simulink model "PhysicalHyperCook"  (R2026a)
settings: Solver=VariableStepAuto  StopTime=14400
undefined symbols (not defined in the file): Fault_T_Cook1, Fault_T_Cook2, Fault_T_Cook3, Fault_T_Cook4, Fault_T_Pack, Fault_T_Prep1, Fault_T_Prep2, Fault_T_QC, HC_PackRate_bph, HC_PrepRate_bph, HC_QCRate_bph, HC_Resupply_bph, Recipe_Block_s, Recipe_Count, Recipe_Flush_s, Resupply_Cutoff_T, Transport_Latency_s, Transport_Rate_bph
(part 1 of 2)
settings Model: DataDictionary=PhysicalHyperCookData.sldd  Creator=sarah  LastModifiedBy=sdagen

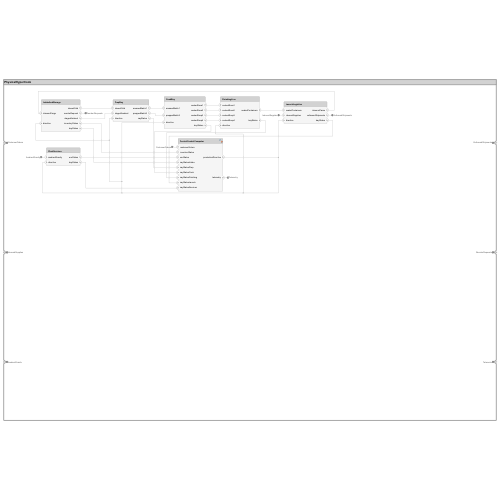
[thumbnail: Simulink's stored preview of the top-level diagram]
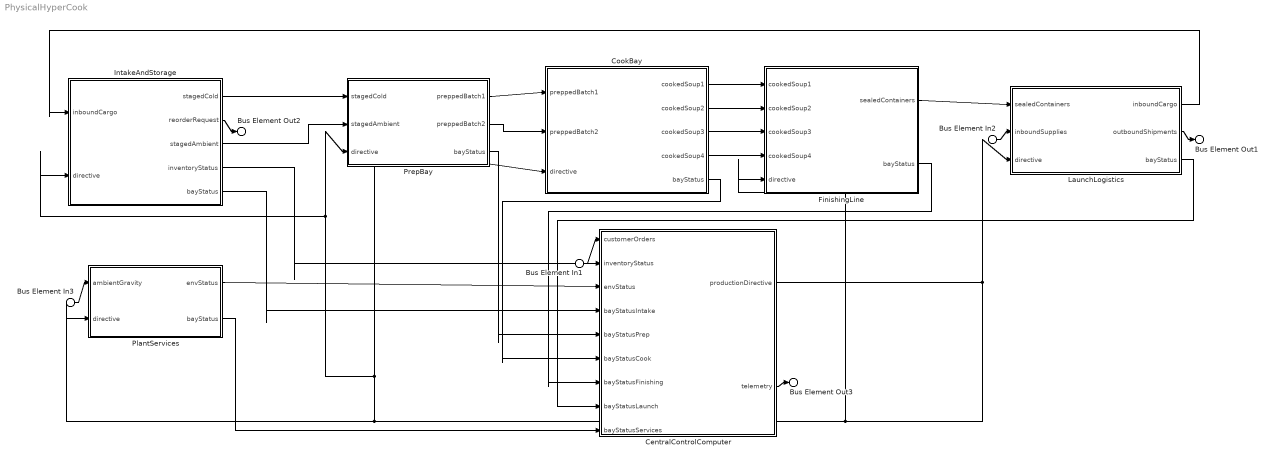
== system PhysicalHyperCook ==
  Bus Element In1 : Inport  PortName=CustomerOrders
  Bus Element In2 : Inport  Port=2  PortName=InboundSupplies
  Bus Element In3 : Inport  Port=3  PortName=AmbientGravity
  CentralControlComputer : Subsystem
      settings: PortSchema="{\"entries\":[{\"content\":{\"headerSize\":26,\"margin\":15,\"minimumSpacing\":25,\"sides\":[{\"content\":{\"connectorIds\":[\"In1\",\"In2\",\"In3\",\"In4\",\"In5\",\"In6\",\"In7\",\"In8\",\"In9\"]},\"type\":\"ConnectorPlacement.EquallySpacedRectSide\",\"uuid\":\"f830f98a-8e8b-4468-adf4-d6eab644987f\"},{\"content\":{\"connectorIds\":[\"Out1\",\"Out2\"],\"side\":\"RIGHT\"},\"type\":\"ConnectorPlacement.EquallySpacedRectSide\",\"uuid\":\"7e0d0116-b3ba-4668-b638-30d0f54ba087\"},{\"content\":{\"side\":\"TOP\"},\"type\":\"ConnectorPlacement.EquallySpacedRectSide\",\"uuid\":\"7b4146d3-46d2-45ca-8c34-b106f0d8cedd\"}]},\"type\":\"ConnectorPlacement.EquallySpacedConnector\",\"uuid\":\"3d911b2d-a78f-42ea-b869-5e09982d9f54\"}],\"packageUris\":[\"http://schema.mathworks.com/mf0/Connector/R2020b\"],\"version\":\"1.0\"}"
  CookBay : Subsystem
      settings: PortSchema="{\"entries\":[{\"content\":{\"headerSize\":26,\"margin\":15,\"minimumSpacing\":25,\"sides\":[{\"content\":{\"connectorIds\":[\"In2\",\"In3\",\"In1\"]},\"type\":\"ConnectorPlacement.EquallySpacedRectSide\",\"uuid\":\"3a94c7fc-0b9e-4df5-a2de-1d2483378dcb\"},{\"content\":{\"connectorIds\":[\"Out1\",\"Out2\",\"Out3\",\"Out4\",\"Out5\"],\"side\":\"RIGHT\"},\"type\":\"ConnectorPlacement.EquallySpacedRectSide\",\"uuid\":\"607e1f04-41cc-4c9a-b401-96cdf33819d0\"},{\"content\":{\"side\":\"TOP\"},\"type\":\"ConnectorPlacement.EquallySpacedRectSide\",\"uuid\":\"2ee07fc7-54c6-4cee-9888-3f37ad01f332\"}]},\"type\":\"ConnectorPlacement.EquallySpacedConnector\",\"uuid\":\"f91f3af9-eaeb-4625-ae6e-5ceb7fb8b64c\"}],\"packageUris\":[\"http://schema.mathworks.com/mf0/Connector/R2020b\"],\"version\":\"1.0\"}"
  FinishingLine : Subsystem
      settings: PortSchema="{\"entries\":[{\"content\":{\"headerSize\":26,\"margin\":15,\"minimumSpacing\":25,\"sides\":[{\"content\":{\"connectorIds\":[\"In2\",\"In3\",\"In4\",\"In5\",\"In1\"]},\"type\":\"ConnectorPlacement.EquallySpacedRectSide\",\"uuid\":\"3a94c7fc-0b9e-4df5-a2de-1d2483378dcb\"},{\"content\":{\"connectorIds\":[\"Out1\",\"Out2\"],\"side\":\"RIGHT\"},\"type\":\"ConnectorPlacement.EquallySpacedRectSide\",\"uuid\":\"607e1f04-41cc-4c9a-b401-96cdf33819d0\"},{\"content\":{\"side\":\"TOP\"},\"type\":\"ConnectorPlacement.EquallySpacedRectSide\",\"uuid\":\"2ee07fc7-54c6-4cee-9888-3f37ad01f332\"}]},\"type\":\"ConnectorPlacement.EquallySpacedConnector\",\"uuid\":\"f91f3af9-eaeb-4625-ae6e-5ceb7fb8b64c\"}],\"packageUris\":[\"http://schema.mathworks.com/mf0/Connector/R2020b\"],\"version\":\"1.0\"}"
  IntakeAndStorage : Subsystem
      settings: PortSchema="{\"entries\":[{\"content\":{\"headerSize\":26,\"margin\":15,\"minimumSpacing\":25,\"sides\":[{\"content\":{\"connectorIds\":[\"In2\",\"In1\"]},\"type\":\"ConnectorPlacement.EquallySpacedRectSide\",\"uuid\":\"3a94c7fc-0b9e-4df5-a2de-1d2483378dcb\"},{\"content\":{\"connectorIds\":[\"Out1\",\"Out2\",\"Out4\",\"Out3\",\"Out5\"],\"side\":\"RIGHT\"},\"type\":\"ConnectorPlacement.EquallySpacedRectSide\",\"uuid\":\"607e1f04-41cc-4c9a-b401-96cdf33819d0\"},{\"content\":{\"side\":\"TOP\"},\"type\":\"ConnectorPlacement.EquallySpacedRectSide\",\"uuid\":\"2ee07fc7-54c6-4cee-9888-3f37ad01f332\"}]},\"type\":\"ConnectorPlacement.EquallySpacedConnector\",\"uuid\":\"f91f3af9-eaeb-4625-ae6e-5ceb7fb8b64c\"}],\"packageUris\":[\"http://schema.mathworks.com/mf0/Connector/R2020b\"],\"version\":\"1.0\"}"
  LaunchLogistics : Subsystem
      settings: PortSchema="{\"entries\":[{\"content\":{\"headerSize\":26,\"margin\":15,\"minimumSpacing\":25,\"sides\":[{\"content\":{\"connectorIds\":[\"In2\",\"In3\",\"In1\"]},\"type\":\"ConnectorPlacement.EquallySpacedRectSide\",\"uuid\":\"3a94c7fc-0b9e-4df5-a2de-1d2483378dcb\"},{\"content\":{\"connectorIds\":[\"Out1\",\"Out2\",\"Out3\"],\"side\":\"RIGHT\"},\"type\":\"ConnectorPlacement.EquallySpacedRectSide\",\"uuid\":\"607e1f04-41cc-4c9a-b401-96cdf33819d0\"},{\"content\":{\"side\":\"TOP\"},\"type\":\"ConnectorPlacement.EquallySpacedRectSide\",\"uuid\":\"2ee07fc7-54c6-4cee-9888-3f37ad01f332\"}]},\"type\":\"ConnectorPlacement.EquallySpacedConnector\",\"uuid\":\"f91f3af9-eaeb-4625-ae6e-5ceb7fb8b64c\"}],\"packageUris\":[\"http://schema.mathworks.com/mf0/Connector/R2020b\"],\"version\":\"1.0\"}"
  PlantServices : Subsystem
      settings: PortSchema="{\"entries\":[{\"content\":{\"headerSize\":26,\"margin\":15,\"minimumSpacing\":25,\"sides\":[{\"content\":{\"connectorIds\":[\"In2\",\"In1\"]},\"type\":\"ConnectorPlacement.EquallySpacedRectSide\",\"uuid\":\"3a94c7fc-0b9e-4df5-a2de-1d2483378dcb\"},{\"content\":{\"connectorIds\":[\"Out1\",\"Out2\"],\"side\":\"RIGHT\"},\"type\":\"ConnectorPlacement.EquallySpacedRectSide\",\"uuid\":\"607e1f04-41cc-4c9a-b401-96cdf33819d0\"},{\"content\":{\"side\":\"TOP\"},\"type\":\"ConnectorPlacement.EquallySpacedRectSide\",\"uuid\":\"2ee07fc7-54c6-4cee-9888-3f37ad01f332\"}]},\"type\":\"ConnectorPlacement.EquallySpacedConnector\",\"uuid\":\"f91f3af9-eaeb-4625-ae6e-5ceb7fb8b64c\"}],\"packageUris\":[\"http://schema.mathworks.com/mf0/Connector/R2020b\"],\"version\":\"1.0\"}"
  PrepBay : Subsystem
      settings: PortSchema="{\"entries\":[{\"content\":{\"headerSize\":26,\"margin\":15,\"minimumSpacing\":25,\"sides\":[{\"content\":{\"connectorIds\":[\"In2\",\"In3\",\"In1\"]},\"type\":\"ConnectorPlacement.EquallySpacedRectSide\",\"uuid\":\"3a94c7fc-0b9e-4df5-a2de-1d2483378dcb\"},{\"content\":{\"connectorIds\":[\"Out1\",\"Out2\",\"Out3\"],\"side\":\"RIGHT\"},\"type\":\"ConnectorPlacement.EquallySpacedRectSide\",\"uuid\":\"607e1f04-41cc-4c9a-b401-96cdf33819d0\"},{\"content\":{\"side\":\"TOP\"},\"type\":\"ConnectorPlacement.EquallySpacedRectSide\",\"uuid\":\"2ee07fc7-54c6-4cee-9888-3f37ad01f332\"}]},\"type\":\"ConnectorPlacement.EquallySpacedConnector\",\"uuid\":\"f91f3af9-eaeb-4625-ae6e-5ceb7fb8b64c\"}],\"packageUris\":[\"http://schema.mathworks.com/mf0/Connector/R2020b\"],\"version\":\"1.0\"}"
  Bus Element Out1 : Outport  PortName=OutboundShipments
  Bus Element Out2 : Outport  Port=2  PortName=ReorderRequests
  Bus Element Out3 : Outport  Port=3  PortName=Telemetry
  wires:
  PrepBay/3(bayStatus) -> CentralControlComputer/5(bayStatusPrep)
  Bus Element In2/1 -> LaunchLogistics/3(inboundSupplies)
  CentralControlComputer/1(productionDirective) -> LaunchLogistics/1(directive), IntakeAndStorage/1(directive), PrepBay/1(directive), CookBay/1(directive), PlantServices/1(directive), FinishingLine/1(directive)
  Bus Element In3/1 -> PlantServices/2(ambientGravity)
  LaunchLogistics/1(inboundCargo) -> IntakeAndStorage/2(inboundCargo)
  LaunchLogistics/2(outboundShipments) -> Bus Element Out1/1
  LaunchLogistics/3(bayStatus) -> CentralControlComputer/8(bayStatusLaunch)
  PrepBay/1(preppedBatch1) -> CookBay/2(preppedBatch1)
  PrepBay/2(preppedBatch2) -> CookBay/3(preppedBatch2)
  FinishingLine/1(sealedContainers) -> LaunchLogistics/2(sealedContainers)
  FinishingLine/2(bayStatus) -> CentralControlComputer/7(bayStatusFinishing)
  IntakeAndStorage/1(stagedCold) -> PrepBay/2(stagedCold)
  IntakeAndStorage/2(reorderRequest) -> Bus Element Out2/1
  IntakeAndStorage/3(inventoryStatus) -> CentralControlComputer/2(inventoryStatus)
  IntakeAndStorage/4(stagedAmbient) -> PrepBay/3(stagedAmbient)
  IntakeAndStorage/5(bayStatus) -> CentralControlComputer/4(bayStatusIntake)
  Bus Element In1/1 -> CentralControlComputer/1(customerOrders)
  CookBay/1(cookedSoup1) -> FinishingLine/2(cookedSoup1)
  CookBay/2(cookedSoup2) -> FinishingLine/3(cookedSoup2)
  CookBay/3(cookedSoup3) -> FinishingLine/4(cookedSoup3)
  CookBay/4(cookedSoup4) -> FinishingLine/5(cookedSoup4)
  CookBay/5(bayStatus) -> CentralControlComputer/6(bayStatusCook)
  PlantServices/2(bayStatus) -> CentralControlComputer/9(bayStatusServices)
  PlantServices/1(envStatus) -> CentralControlComputer/3(envStatus)
  CentralControlComputer/2(telemetry) -> Bus Element Out3/1

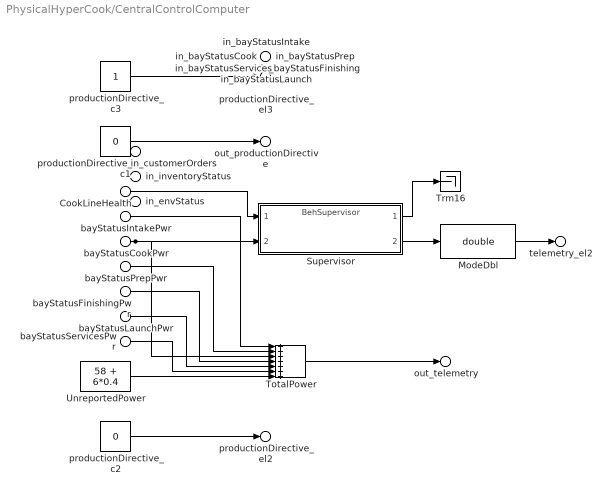
== system PhysicalHyperCook/CentralControlComputer ==
  in_customerOrders : Inport  PortName=customerOrders
  in_inventoryStatus : Inport  Port=2  PortName=inventoryStatus
  in_envStatus : Inport  Port=3  PortName=envStatus
  in_bayStatusIntake : Inport  Port=4  PortName=bayStatusIntake
  bayStatusIntakePwr : Inport  Port=4  PortName=bayStatusIntake  Element=power_kW
  in_bayStatusPrep : Inport  Port=5  PortName=bayStatusPrep
  bayStatusPrepPwr : Inport  Port=5  PortName=bayStatusPrep  Element=power_kW
  in_bayStatusCook : Inport  Port=6  PortName=bayStatusCook  Element=power_kW
  bayStatusCookPwr : Inport  Port=6  PortName=bayStatusCook  Element=power_kW
  CookLineHealth : Inport  Port=6  PortName=bayStatusCook  Element=lineHealth
  in_bayStatusFinishing : Inport  Port=7  PortName=bayStatusFinishing
  bayStatusFinishingPwr : Inport  Port=7  PortName=bayStatusFinishing  Element=power_kW
  in_bayStatusLaunch : Inport  Port=8  PortName=bayStatusLaunch
  bayStatusLaunchPwr : Inport  Port=8  PortName=bayStatusLaunch  Element=power_kW
  in_bayStatusServices : Inport  Port=9  PortName=bayStatusServices
  bayStatusServicesPwr : Inport  Port=9  PortName=bayStatusServices  Element=power_kW
  ModeDbl : DataTypeConversion  OutDataTypeStr=double  SaturateOnIntegerOverflow=off  RndMeth=Floor
  Supervisor : ModelReference  ModelNameDialog=BehSupervisor  ParameterArgumentNames=NumLines  ParameterArgumentValues=HC_NumLines  UsingDefaultArgumentValue=0  SimulationMode=Normal  ModelReferenceVersion=1.8
  TotalPower : Sum  Inputs=+++++++
  Trm16 : Terminator
  UnreportedPower : Constant  Value=58 + 6*0.4
  productionDirective_c1 : Constant  Value=0
  productionDirective_c2 : Constant  Value=0
  productionDirective_c3 : Constant
  out_productionDirective : Outport  PortName=productionDirective  Element=cmdType
  productionDirective_el2 : Outport  PortName=productionDirective  Element=targetId
  productionDirective_el3 : Outport  PortName=productionDirective  Element=setpoint
  out_telemetry : Outport  Port=2  PortName=telemetry  Element=totalPower_kW
  telemetry_el2 : Outport  Port=2  PortName=telemetry  Element=plantMode
  wires:
  productionDirective_c3/1 -> productionDirective_el3/1
  bayStatusPrepPwr/1 -> TotalPower/2
  CookLineHealth/1 -> Supervisor/1
  productionDirective_c1/1 -> out_productionDirective/1
  bayStatusIntakePwr/1 -> TotalPower/1
  bayStatusLaunchPwr/1 -> TotalPower/5
  bayStatusCookPwr/1 -> Supervisor/2, TotalPower/3
  bayStatusFinishingPwr/1 -> TotalPower/4
  Supervisor/2 -> ModeDbl/1
  bayStatusServicesPwr/1 -> TotalPower/6
  UnreportedPower/1 -> TotalPower/7
  productionDirective_c2/1 -> productionDirective_el2/1
  Supervisor/1 -> Trm16/1
  TotalPower/1 -> out_telemetry/1
  ModeDbl/1 -> telemetry_el2/1

== system PhysicalHyperCook/CookBay ==
  Bus Element In1 : Inport  PortName=directive
  Bus Element In3 : Inport  Port=2  PortName=preppedBatch1
  Bus Element In4 : Inport  Port=3  PortName=preppedBatch2
  ContinuousCookLine1 : Subsystem
      settings: PortSchema="{\"entries\":[{\"content\":{\"headerSize\":26,\"margin\":15,\"minimumSpacing\":25,\"sides\":[{\"content\":{\"connectorIds\":[\"In1\",\"In2\"]},\"type\":\"ConnectorPlacement.EquallySpacedRectSide\",\"uuid\":\"f830f98a-8e8b-4468-adf4-d6eab644987f\"},{\"content\":{\"connectorIds\":[\"Out1\",\"Out2\"],\"side\":\"RIGHT\"},\"type\":\"ConnectorPlacement.EquallySpacedRectSide\",\"uuid\":\"7e0d0116-b3ba-4668-b638-30d0f54ba087\"},{\"content\":{\"side\":\"TOP\"},\"type\":\"ConnectorPlacement.EquallySpacedRectSide\",\"uuid\":\"7b4146d3-46d2-45ca-8c34-b106f0d8cedd\"}]},\"type\":\"ConnectorPlacement.EquallySpacedConnector\",\"uuid\":\"3d911b2d-a78f-42ea-b869-5e09982d9f54\"}],\"packageUris\":[\"http://schema.mathworks.com/mf0/Connector/R2020b\"],\"version\":\"1.0\"}"
  ContinuousCookLine2 : Subsystem
      settings: PortSchema="{\"entries\":[{\"content\":{\"headerSize\":26,\"margin\":15,\"minimumSpacing\":25,\"sides\":[{\"content\":{\"connectorIds\":[\"In1\",\"In2\"]},\"type\":\"ConnectorPlacement.EquallySpacedRectSide\",\"uuid\":\"f830f98a-8e8b-4468-adf4-d6eab644987f\"},{\"content\":{\"connectorIds\":[\"Out1\",\"Out2\"],\"side\":\"RIGHT\"},\"type\":\"ConnectorPlacement.EquallySpacedRectSide\",\"uuid\":\"7e0d0116-b3ba-4668-b638-30d0f54ba087\"},{\"content\":{\"side\":\"TOP\"},\"type\":\"ConnectorPlacement.EquallySpacedRectSide\",\"uuid\":\"7b4146d3-46d2-45ca-8c34-b106f0d8cedd\"}]},\"type\":\"ConnectorPlacement.EquallySpacedConnector\",\"uuid\":\"3d911b2d-a78f-42ea-b869-5e09982d9f54\"}],\"packageUris\":[\"http://schema.mathworks.com/mf0/Connector/R2020b\"],\"version\":\"1.0\"}"
  ContinuousCookLine3 : Subsystem
      settings: PortSchema="{\"entries\":[{\"content\":{\"headerSize\":26,\"margin\":15,\"minimumSpacing\":25,\"sides\":[{\"content\":{\"connectorIds\":[\"In1\",\"In2\"]},\"type\":\"ConnectorPlacement.EquallySpacedRectSide\",\"uuid\":\"f830f98a-8e8b-4468-adf4-d6eab644987f\"},{\"content\":{\"connectorIds\":[\"Out1\",\"Out2\"],\"side\":\"RIGHT\"},\"type\":\"ConnectorPlacement.EquallySpacedRectSide\",\"uuid\":\"7e0d0116-b3ba-4668-b638-30d0f54ba087\"},{\"content\":{\"side\":\"TOP\"},\"type\":\"ConnectorPlacement.EquallySpacedRectSide\",\"uuid\":\"7b4146d3-46d2-45ca-8c34-b106f0d8cedd\"}]},\"type\":\"ConnectorPlacement.EquallySpacedConnector\",\"uuid\":\"3d911b2d-a78f-42ea-b869-5e09982d9f54\"}],\"packageUris\":[\"http://schema.mathworks.com/mf0/Connector/R2020b\"],\"version\":\"1.0\"}"
  ContinuousCookLine4 : Subsystem
      settings: PortSchema="{\"entries\":[{\"content\":{\"headerSize\":26,\"margin\":15,\"minimumSpacing\":25,\"sides\":[{\"content\":{\"connectorIds\":[\"In1\",\"In2\"]},\"type\":\"ConnectorPlacement.EquallySpacedRectSide\",\"uuid\":\"f830f98a-8e8b-4468-adf4-d6eab644987f\"},{\"content\":{\"connectorIds\":[\"Out1\",\"Out2\"],\"side\":\"RIGHT\"},\"type\":\"ConnectorPlacement.EquallySpacedRectSide\",\"uuid\":\"7e0d0116-b3ba-4668-b638-30d0f54ba087\"},{\"content\":{\"side\":\"TOP\"},\"type\":\"ConnectorPlacement.EquallySpacedRectSide\",\"uuid\":\"7b4146d3-46d2-45ca-8c34-b106f0d8cedd\"}]},\"type\":\"ConnectorPlacement.EquallySpacedConnector\",\"uuid\":\"3d911b2d-a78f-42ea-b869-5e09982d9f54\"}],\"packageUris\":[\"http://schema.mathworks.com/mf0/Connector/R2020b\"],\"version\":\"1.0\"}"
  CookController : Subsystem
      settings: PortSchema="{\"entries\":[{\"content\":{\"headerSize\":26,\"margin\":15,\"minimumSpacing\":25,\"sides\":[{\"content\":{\"connectorIds\":[\"In1\",\"In2\",\"In3\",\"In4\",\"In5\"]},\"type\":\"ConnectorPlacement.EquallySpacedRectSide\",\"uuid\":\"0731d988-4a26-4db6-8347-b78d2aa6954f\"},{\"content\":{\"connectorIds\":[\"Out1\",\"Out2\"],\"side\":\"RIGHT\"},\"type\":\"ConnectorPlacement.EquallySpacedRectSide\",\"uuid\":\"6e8ac7ed-a816-4c7e-8f31-c61224c9ac03\"},{\"content\":{\"side\":\"TOP\"},\"type\":\"ConnectorPlacement.EquallySpacedRectSide\",\"uuid\":\"7c48a918-2743-4697-bc21-ce4fb8bbcea2\"}]},\"type\":\"ConnectorPlacement.EquallySpacedConnector\",\"uuid\":\"5e30be34-c1af-4919-9af8-d4df8145ecd1\"}],\"packageUris\":[\"http://schema.mathworks.com/mf0/Connector/R2020b\"],\"version\":\"1.0\"}"
  Bus Element Out5 : Outport  PortName=cookedSoup1
  Bus Element Out6 : Outport  Port=2  PortName=cookedSoup2
  Bus Element Out7 : Outport  Port=3  PortName=cookedSoup3
  Bus Element Out8 : Outport  Port=4  PortName=cookedSoup4
  Bus Element Out9 : Outport  Port=5  PortName=bayStatus
  wires:
  Bus Element In1/1 -> CookController/1(directive)
  CookController/2(bayStatus) -> Bus Element Out9/1
  ContinuousCookLine4/2(statusCook4) -> CookController/5(statusCook4)
  Bus Element In3/1 -> ContinuousCookLine1/1(preppedBatch1), ContinuousCookLine2/1(preppedBatch1)
  CookController/1(bayDirective) -> ContinuousCookLine1/2(directive), ContinuousCookLine3/2(directive), ContinuousCookLine2/2(directive), ContinuousCookLine4/2(directive)
  Bus Element In4/1 -> ContinuousCookLine4/1(preppedBatch2), ContinuousCookLine3/1(preppedBatch2)
  ContinuousCookLine4/1(cookedSoup4) -> Bus Element Out8/1
  ContinuousCookLine2/1(cookedSoup2) -> Bus Element Out6/1
  ContinuousCookLine2/2(statusCook2) -> CookController/3(statusCook2)
  ContinuousCookLine1/1(cookedSoup1) -> Bus Element Out5/1
  ContinuousCookLine1/2(statusCook1) -> CookController/2(statusCook1)
  ContinuousCookLine3/1(cookedSoup3) -> Bus Element Out7/1
  ContinuousCookLine3/2(statusCook3) -> CookController/4(statusCook3)

== system PhysicalHyperCook/FinishingLine ==
  Bus Element In1 : Inport  PortName=directive
  Bus Element In3 : Inport  Port=2  PortName=cookedSoup1
  Bus Element In4 : Inport  Port=3  PortName=cookedSoup2
  Bus Element In5 : Inport  Port=4  PortName=cookedSoup3
  Bus Element In6 : Inport  Port=5  PortName=cookedSoup4
  FinishingController : Subsystem
      settings: PortSchema="{\"entries\":[{\"content\":{\"headerSize\":26,\"margin\":15,\"minimumSpacing\":25,\"sides\":[{\"content\":{\"connectorIds\":[\"In1\",\"In2\",\"In3\"]},\"type\":\"ConnectorPlacement.EquallySpacedRectSide\",\"uuid\":\"0731d988-4a26-4db6-8347-b78d2aa6954f\"},{\"content\":{\"connectorIds\":[\"Out1\",\"Out2\"],\"side\":\"RIGHT\"},\"type\":\"ConnectorPlacement.EquallySpacedRectSide\",\"uuid\":\"6e8ac7ed-a816-4c7e-8f31-c61224c9ac03\"},{\"content\":{\"side\":\"TOP\"},\"type\":\"ConnectorPlacement.EquallySpacedRectSide\",\"uuid\":\"7c48a918-2743-4697-bc21-ce4fb8bbcea2\"}]},\"type\":\"ConnectorPlacement.EquallySpacedConnector\",\"uuid\":\"5e30be34-c1af-4919-9af8-d4df8145ecd1\"}],\"packageUris\":[\"http://schema.mathworks.com/mf0/Connector/R2020b\"],\"version\":\"1.0\"}"
  HighSpeedPackagingLine : Subsystem
      settings: PortSchema="{\"entries\":[{\"content\":{\"headerSize\":26,\"margin\":15,\"minimumSpacing\":25,\"sides\":[{\"content\":{\"connectorIds\":[\"In1\",\"In2\"]},\"type\":\"ConnectorPlacement.EquallySpacedRectSide\",\"uuid\":\"f830f98a-8e8b-4468-adf4-d6eab644987f\"},{\"content\":{\"connectorIds\":[\"Out1\",\"Out2\"],\"side\":\"RIGHT\"},\"type\":\"ConnectorPlacement.EquallySpacedRectSide\",\"uuid\":\"7e0d0116-b3ba-4668-b638-30d0f54ba087\"},{\"content\":{\"side\":\"TOP\"},\"type\":\"ConnectorPlacement.EquallySpacedRectSide\",\"uuid\":\"7b4146d3-46d2-45ca-8c34-b106f0d8cedd\"}]},\"type\":\"ConnectorPlacement.EquallySpacedConnector\",\"uuid\":\"3d911b2d-a78f-42ea-b869-5e09982d9f54\"}],\"packageUris\":[\"http://schema.mathworks.com/mf0/Connector/R2020b\"],\"version\":\"1.0\"}"
  InlineQCScanner : Subsystem
      settings: PortSchema="{\"entries\":[{\"content\":{\"headerSize\":26,\"margin\":15,\"minimumSpacing\":25,\"sides\":[{\"content\":{\"connectorIds\":[\"In1\",\"In2\",\"In3\",\"In4\",\"In5\"]},\"type\":\"ConnectorPlacement.EquallySpacedRectSide\",\"uuid\":\"f830f98a-8e8b-4468-adf4-d6eab644987f\"},{\"content\":{\"connectorIds\":[\"Out1\",\"Out2\"],\"side\":\"RIGHT\"},\"type\":\"ConnectorPlacement.EquallySpacedRectSide\",\"uuid\":\"7e0d0116-b3ba-4668-b638-30d0f54ba087\"},{\"content\":{\"side\":\"TOP\"},\"type\":\"ConnectorPlacement.EquallySpacedRectSide\",\"uuid\":\"7b4146d3-46d2-45ca-8c34-b106f0d8cedd\"}]},\"type\":\"ConnectorPlacement.EquallySpacedConnector\",\"uuid\":\"3d911b2d-a78f-42ea-b869-5e09982d9f54\"}],\"packageUris\":[\"http://schema.mathworks.com/mf0/Connector/R2020b\"],\"version\":\"1.0\"}"
  Bus Element Out1 : Outport  PortName=sealedContainers
  Bus Element Out4 : Outport  Port=2  PortName=bayStatus
  wires:
  Bus Element In3/1 -> InlineQCScanner/1(cookedSoup1)
  Bus Element In4/1 -> InlineQCScanner/2(cookedSoup2)
  Bus Element In5/1 -> InlineQCScanner/3(cookedSoup3)
  Bus Element In6/1 -> InlineQCScanner/4(cookedSoup4)
  HighSpeedPackagingLine/2(statusPack) -> FinishingController/2(statusPack)
  InlineQCScanner/1(approvedSoup) -> HighSpeedPackagingLine/1(approvedSoup)
  HighSpeedPackagingLine/1(sealedContainers) -> Bus Element Out1/1
  InlineQCScanner/2(statusQA) -> FinishingController/3(statusQA)
  Bus Element In1/1 -> FinishingController/1(directive)
  FinishingController/1(bayDirective) -> InlineQCScanner/5(directive), HighSpeedPackagingLine/2(directive)
  FinishingController/2(bayStatus) -> Bus Element Out4/1

== system PhysicalHyperCook/IntakeAndStorage ==
  Bus Element In1 : Inport  PortName=directive
  Bus Element In2 : Inport  Port=2  PortName=inboundCargo
  AmbientStorageSilo : Subsystem
      settings: PortSchema="{\"entries\":[{\"content\":{\"headerSize\":26,\"margin\":15,\"minimumSpacing\":25,\"sides\":[{\"content\":{\"connectorIds\":[\"In1\",\"In2\"]},\"type\":\"ConnectorPlacement.EquallySpacedRectSide\",\"uuid\":\"f830f98a-8e8b-4468-adf4-d6eab644987f\"},{\"content\":{\"connectorIds\":[\"Out1\",\"Out2\",\"Out3\"],\"side\":\"RIGHT\"},\"type\":\"ConnectorPlacement.EquallySpacedRectSide\",\"uuid\":\"7e0d0116-b3ba-4668-b638-30d0f54ba087\"},{\"content\":{\"side\":\"TOP\"},\"type\":\"ConnectorPlacement.EquallySpacedRectSide\",\"uuid\":\"7b4146d3-46d2-45ca-8c34-b106f0d8cedd\"}]},\"type\":\"ConnectorPlacement.EquallySpacedConnector\",\"uuid\":\"3d911b2d-a78f-42ea-b869-5e09982d9f54\"}],\"packageUris\":[\"http://schema.mathworks.com/mf0/Connector/R2020b\"],\"version\":\"1.0\"}"
  CargoGantryDock : Subsystem
      settings: PortSchema="{\"entries\":[{\"content\":{\"headerSize\":26,\"margin\":15,\"minimumSpacing\":25,\"sides\":[{\"content\":{\"connectorIds\":[\"In1\",\"In2\"]},\"type\":\"ConnectorPlacement.EquallySpacedRectSide\",\"uuid\":\"f830f98a-8e8b-4468-adf4-d6eab644987f\"},{\"content\":{\"connectorIds\":[\"Out1\",\"Out2\"],\"side\":\"RIGHT\"},\"type\":\"ConnectorPlacement.EquallySpacedRectSide\",\"uuid\":\"7e0d0116-b3ba-4668-b638-30d0f54ba087\"},{\"content\":{\"side\":\"TOP\"},\"type\":\"ConnectorPlacement.EquallySpacedRectSide\",\"uuid\":\"7b4146d3-46d2-45ca-8c34-b106f0d8cedd\"}]},\"type\":\"ConnectorPlacement.EquallySpacedConnector\",\"uuid\":\"3d911b2d-a78f-42ea-b869-5e09982d9f54\"}],\"packageUris\":[\"http://schema.mathworks.com/mf0/Connector/R2020b\"],\"version\":\"1.0\"}"
  ColdStorageVault : Subsystem
      settings: PortSchema="{\"entries\":[{\"content\":{\"headerSize\":26,\"margin\":15,\"minimumSpacing\":25,\"sides\":[{\"content\":{\"connectorIds\":[\"In1\",\"In2\"]},\"type\":\"ConnectorPlacement.EquallySpacedRectSide\",\"uuid\":\"f830f98a-8e8b-4468-adf4-d6eab644987f\"},{\"content\":{\"connectorIds\":[\"Out1\",\"Out2\",\"Out3\"],\"side\":\"RIGHT\"},\"type\":\"ConnectorPlacement.EquallySpacedRectSide\",\"uuid\":\"7e0d0116-b3ba-4668-b638-30d0f54ba087\"},{\"content\":{\"side\":\"TOP\"},\"type\":\"ConnectorPlacement.EquallySpacedRectSide\",\"uuid\":\"7b4146d3-46d2-45ca-8c34-b106f0d8cedd\"}]},\"type\":\"ConnectorPlacement.EquallySpacedConnector\",\"uuid\":\"3d911b2d-a78f-42ea-b869-5e09982d9f54\"}],\"packageUris\":[\"http://schema.mathworks.com/mf0/Connector/R2020b\"],\"version\":\"1.0\"}"
  IntakeController : Subsystem
      settings: PortSchema="{\"entries\":[{\"content\":{\"headerSize\":26,\"margin\":15,\"minimumSpacing\":25,\"sides\":[{\"content\":{\"connectorIds\":[\"In1\",\"In2\",\"In3\",\"In4\"]},\"type\":\"ConnectorPlacement.EquallySpacedRectSide\",\"uuid\":\"0731d988-4a26-4db6-8347-b78d2aa6954f\"},{\"content\":{\"connectorIds\":[\"Out1\",\"Out2\"],\"side\":\"RIGHT\"},\"type\":\"ConnectorPlacement.EquallySpacedRectSide\",\"uuid\":\"6e8ac7ed-a816-4c7e-8f31-c61224c9ac03\"},{\"content\":{\"side\":\"TOP\"},\"type\":\"ConnectorPlacement.EquallySpacedRectSide\",\"uuid\":\"7c48a918-2743-4697-bc21-ce4fb8bbcea2\"}]},\"type\":\"ConnectorPlacement.EquallySpacedConnector\",\"uuid\":\"5e30be34-c1af-4919-9af8-d4df8145ecd1\"}],\"packageUris\":[\"http://schema.mathworks.com/mf0/Connector/R2020b\"],\"version\":\"1.0\"}"
  InventorySensorGrid : Subsystem
      settings: PortSchema="{\"entries\":[{\"content\":{\"headerSize\":26,\"margin\":15,\"minimumSpacing\":25,\"sides\":[{\"content\":{\"connectorIds\":[\"In1\",\"In2\"]},\"type\":\"ConnectorPlacement.EquallySpacedRectSide\",\"uuid\":\"f830f98a-8e8b-4468-adf4-d6eab644987f\"},{\"content\":{\"connectorIds\":[\"Out1\",\"Out2\"],\"side\":\"RIGHT\"},\"type\":\"ConnectorPlacement.EquallySpacedRectSide\",\"uuid\":\"7e0d0116-b3ba-4668-b638-30d0f54ba087\"},{\"content\":{\"side\":\"TOP\"},\"type\":\"ConnectorPlacement.EquallySpacedRectSide\",\"uuid\":\"7b4146d3-46d2-45ca-8c34-b106f0d8cedd\"}]},\"type\":\"ConnectorPlacement.EquallySpacedConnector\",\"uuid\":\"3d911b2d-a78f-42ea-b869-5e09982d9f54\"}],\"packageUris\":[\"http://schema.mathworks.com/mf0/Connector/R2020b\"],\"version\":\"1.0\"}"
  Bus Element Out1 : Outport  PortName=stagedCold
  Bus Element Out2 : Outport  Port=2  PortName=reorderRequest
  Bus Element Out3 : Outport  Port=3  PortName=inventoryStatus
  Bus Element Out7 : Outport  Port=4  PortName=stagedAmbient
  Bus Element Out8 : Outport  Port=5  PortName=bayStatus
  wires:
  ColdStorageVault/1(stagedCold) -> Bus Element Out1/1
  IntakeController/1(bayDirective) -> AmbientStorageSilo/2(directive), ColdStorageVault/2(directive), CargoGantryDock/2(directive)
  Bus Element In1/1 -> IntakeController/1(directive)
  AmbientStorageSilo/2(stockAmbient) -> InventorySensorGrid/2(stockAmbient)
  Bus Element In2/1 -> CargoGantryDock/1(inboundCargo)
  CargoGantryDock/2(statusReceive) -> IntakeController/3(statusReceive)
  IntakeController/2(bayStatus) -> Bus Element Out8/1
  CargoGantryDock/1(receivedIngredients) -> ColdStorageVault/1(receivedIngredients), AmbientStorageSilo/1(receivedIngredients)
  AmbientStorageSilo/1(stagedAmbient) -> Bus Element Out7/1
  AmbientStorageSilo/3(statusAmbStore) -> IntakeController/2(statusAmbStore)
  ColdStorageVault/3(statusColdStore) -> IntakeController/4(statusColdStore)
  ColdStorageVault/2(stockCold) -> InventorySensorGrid/1(stockCold)
  InventorySensorGrid/1(inventoryStatus) -> Bus Element Out3/1
  InventorySensorGrid/2(reorderRequest) -> Bus Element Out2/1

== system PhysicalHyperCook/LaunchLogistics ==
  Bus Element In1 : Inport  PortName=directive
  Bus Element In2 : Inport  Port=2  PortName=sealedContainers
  Bus Element In4 : Inport  Port=3  PortName=inboundSupplies
  CargoLoaderGantry : Subsystem
      settings: PortSchema="{\"entries\":[{\"content\":{\"headerSize\":26,\"margin\":15,\"minimumSpacing\":25,\"sides\":[{\"content\":{\"connectorIds\":[\"In1\",\"In2\"]},\"type\":\"ConnectorPlacement.EquallySpacedRectSide\",\"uuid\":\"f830f98a-8e8b-4468-adf4-d6eab644987f\"},{\"content\":{\"connectorIds\":[\"Out1\",\"Out2\",\"Out3\"],\"side\":\"RIGHT\"},\"type\":\"ConnectorPlacement.EquallySpacedRectSide\",\"uuid\":\"7e0d0116-b3ba-4668-b638-30d0f54ba087\"},{\"content\":{\"side\":\"TOP\"},\"type\":\"ConnectorPlacement.EquallySpacedRectSide\",\"uuid\":\"7b4146d3-46d2-45ca-8c34-b106f0d8cedd\"}]},\"type\":\"ConnectorPlacement.EquallySpacedConnector\",\"uuid\":\"3d911b2d-a78f-42ea-b869-5e09982d9f54\"}],\"packageUris\":[\"http://schema.mathworks.com/mf0/Connector/R2020b\"],\"version\":\"1.0\"}"
  LaunchController : Subsystem
      settings: PortSchema="{\"entries\":[{\"content\":{\"headerSize\":26,\"margin\":15,\"minimumSpacing\":25,\"sides\":[{\"content\":{\"connectorIds\":[\"In1\",\"In2\",\"In3\",\"In4\"]},\"type\":\"ConnectorPlacement.EquallySpacedRectSide\",\"uuid\":\"0731d988-4a26-4db6-8347-b78d2aa6954f\"},{\"content\":{\"connectorIds\":[\"Out1\",\"Out2\"],\"side\":\"RIGHT\"},\"type\":\"ConnectorPlacement.EquallySpacedRectSide\",\"uuid\":\"6e8ac7ed-a816-4c7e-8f31-c61224c9ac03\"},{\"content\":{\"side\":\"TOP\"},\"type\":\"ConnectorPlacement.EquallySpacedRectSide\",\"uuid\":\"7c48a918-2743-4697-bc21-ce4fb8bbcea2\"}]},\"type\":\"ConnectorPlacement.EquallySpacedConnector\",\"uuid\":\"5e30be34-c1af-4919-9af8-d4df8145ecd1\"}],\"packageUris\":[\"http://schema.mathworks.com/mf0/Connector/R2020b\"],\"version\":\"1.0\"}"
  LaunchPadComplex : Subsystem
      settings: PortSchema="{\"entries\":[{\"content\":{\"headerSize\":26,\"margin\":15,\"minimumSpacing\":25,\"sides\":[{\"content\":{\"connectorIds\":[\"In1\",\"In2\",\"In3\",\"In4\"]},\"type\":\"ConnectorPlacement.EquallySpacedRectSide\",\"uuid\":\"f830f98a-8e8b-4468-adf4-d6eab644987f\"},{\"content\":{\"connectorIds\":[\"Out1\",\"Out2\",\"Out3\"],\"side\":\"RIGHT\"},\"type\":\"ConnectorPlacement.EquallySpacedRectSide\",\"uuid\":\"7e0d0116-b3ba-4668-b638-30d0f54ba087\"},{\"content\":{\"side\":\"TOP\"},\"type\":\"ConnectorPlacement.EquallySpacedRectSide\",\"uuid\":\"7b4146d3-46d2-45ca-8c34-b106f0d8cedd\"}]},\"type\":\"ConnectorPlacement.EquallySpacedConnector\",\"uuid\":\"3d911b2d-a78f-42ea-b869-5e09982d9f54\"}],\"packageUris\":[\"http://schema.mathworks.com/mf0/Connector/R2020b\"],\"version\":\"1.0\"}"
  RefuelingStation : Subsystem
      settings: PortSchema="{\"entries\":[{\"content\":{\"headerSize\":26,\"margin\":15,\"minimumSpacing\":25,\"sides\":[{\"content\":{\"connectorIds\":[\"In1\"]},\"type\":\"ConnectorPlacement.EquallySpacedRectSide\",\"uuid\":\"f830f98a-8e8b-4468-adf4-d6eab644987f\"},{\"content\":{\"connectorIds\":[\"Out1\"],\"side\":\"RIGHT\"},\"type\":\"ConnectorPlacement.EquallySpacedRectSide\",\"uuid\":\"7e0d0116-b3ba-4668-b638-30d0f54ba087\"},{\"content\":{\"side\":\"TOP\"},\"type\":\"ConnectorPlacement.EquallySpacedRectSide\",\"uuid\":\"7b4146d3-46d2-45ca-8c34-b106f0d8cedd\"}]},\"type\":\"ConnectorPlacement.EquallySpacedConnector\",\"uuid\":\"3d911b2d-a78f-42ea-b869-5e09982d9f54\"}],\"packageUris\":[\"http://schema.mathworks.com/mf0/Connector/R2020b\"],\"version\":\"1.0\"}"
  Bus Element Out1 : Outport  PortName=inboundCargo
  Bus Element Out5 : Outport  Port=2  PortName=outboundShipments
  Bus Element Out6 : Outport  Port=3  PortName=bayStatus
  wires:
  LaunchPadComplex/2(outboundShipments) -> Bus Element Out5/1
  LaunchController/1(bayDirective) -> RefuelingStation/1(directive), CargoLoaderGantry/2(directive), LaunchPadComplex/3(directive)
  Bus Element In4/1 -> LaunchPadComplex/4(inboundSupplies)
  Bus Element In2/1 -> CargoLoaderGantry/1(sealedContainers)
  RefuelingStation/1(statusRefuel) -> LaunchController/4(statusRefuel)
  LaunchPadComplex/1(inboundCargo) -> Bus Element Out1/1
  LaunchPadComplex/3(statusFleet) -> LaunchController/3(statusFleet)
  Bus Element In1/1 -> LaunchController/1(directive)
  LaunchController/2(bayStatus) -> Bus Element Out6/1
  CargoLoaderGantry/1(loadedShipment) -> LaunchPadComplex/1(loadedShipment)
  CargoLoaderGantry/2(manifest) -> LaunchPadComplex/2(manifest)
  CargoLoaderGantry/3(statusDispatch) -> LaunchController/2(statusDispatch)

== system PhysicalHyperCook/PlantServices ==
  Bus Element In2 : Inport  PortName=directive
  Bus Element In4 : Inport  PortName=directive
  Bus Element In3 : Inport  Port=2  PortName=ambientGravity
  ConveyorNetwork : Subsystem
      settings: PortSchema="{\"entries\":[{\"content\":{\"headerSize\":26,\"margin\":15,\"minimumSpacing\":25,\"sides\":[{\"content\":{\"connectorIds\":[\"In1\"]},\"type\":\"ConnectorPlacement.EquallySpacedRectSide\",\"uuid\":\"f830f98a-8e8b-4468-adf4-d6eab644987f\"},{\"content\":{\"connectorIds\":[\"Out1\"],\"side\":\"RIGHT\"},\"type\":\"ConnectorPlacement.EquallySpacedRectSide\",\"uuid\":\"7e0d0116-b3ba-4668-b638-30d0f54ba087\"},{\"content\":{\"side\":\"TOP\"},\"type\":\"ConnectorPlacement.EquallySpacedRectSide\",\"uuid\":\"7b4146d3-46d2-45ca-8c34-b106f0d8cedd\"}]},\"type\":\"ConnectorPlacement.EquallySpacedConnector\",\"uuid\":\"3d911b2d-a78f-42ea-b869-5e09982d9f54\"}],\"packageUris\":[\"http://schema.mathworks.com/mf0/Connector/R2020b\"],\"version\":\"1.0\"}"
  FusionPowerPlant : Subsystem
      settings: PortSchema="{\"entries\":[{\"content\":{\"headerSize\":26,\"margin\":15,\"minimumSpacing\":25,\"sides\":[{\"content\":{\"connectorIds\":[\"In1\"]},\"type\":\"ConnectorPlacement.EquallySpacedRectSide\",\"uuid\":\"f830f98a-8e8b-4468-adf4-d6eab644987f\"},{\"content\":{\"connectorIds\":[\"Out1\"],\"side\":\"RIGHT\"},\"type\":\"ConnectorPlacement.EquallySpacedRectSide\",\"uuid\":\"7e0d0116-b3ba-4668-b638-30d0f54ba087\"},{\"content\":{\"side\":\"TOP\"},\"type\":\"ConnectorPlacement.EquallySpacedRectSide\",\"uuid\":\"7b4146d3-46d2-45ca-8c34-b106f0d8cedd\"}]},\"type\":\"ConnectorPlacement.EquallySpacedConnector\",\"uuid\":\"3d911b2d-a78f-42ea-b869-5e09982d9f54\"}],\"packageUris\":[\"http://schema.mathworks.com/mf0/Connector/R2020b\"],\"version\":\"1.0\"}"
  GravityCompensatorArray : Subsystem
      settings: PortSchema="{\"entries\":[{\"content\":{\"headerSize\":26,\"margin\":15,\"minimumSpacing\":25,\"sides\":[{\"content\":{\"connectorIds\":[\"In1\"]},\"type\":\"ConnectorPlacement.EquallySpacedRectSide\",\"uuid\":\"f830f98a-8e8b-4468-adf4-d6eab644987f\"},{\"content\":{\"connectorIds\":[\"Out1\"],\"side\":\"RIGHT\"},\"type\":\"ConnectorPlacement.EquallySpacedRectSide\",\"uuid\":\"7e0d0116-b3ba-4668-b638-30d0f54ba087\"},{\"content\":{\"side\":\"TOP\"},\"type\":\"ConnectorPlacement.EquallySpacedRectSide\",\"uuid\":\"7b4146d3-46d2-45ca-8c34-b106f0d8cedd\"}]},\"type\":\"ConnectorPlacement.EquallySpacedConnector\",\"uuid\":\"3d911b2d-a78f-42ea-b869-5e09982d9f54\"}],\"packageUris\":[\"http://schema.mathworks.com/mf0/Connector/R2020b\"],\"version\":\"1.0\"}"
  ServicesController : Subsystem
      settings: PortSchema="{\"entries\":[{\"content\":{\"headerSize\":26,\"margin\":15,\"minimumSpacing\":25,\"sides\":[{\"content\":{\"connectorIds\":[\"In1\",\"In2\",\"In3\"]},\"type\":\"ConnectorPlacement.EquallySpacedRectSide\",\"uuid\":\"0731d988-4a26-4db6-8347-b78d2aa6954f\"},{\"content\":{\"connectorIds\":[\"Out1\",\"Out2\"],\"side\":\"RIGHT\"},\"type\":\"ConnectorPlacement.EquallySpacedRectSide\",\"uuid\":\"6e8ac7ed-a816-4c7e-8f31-c61224c9ac03\"},{\"content\":{\"side\":\"TOP\"},\"type\":\"ConnectorPlacement.EquallySpacedRectSide\",\"uuid\":\"7c48a918-2743-4697-bc21-ce4fb8bbcea2\"}]},\"type\":\"ConnectorPlacement.EquallySpacedConnector\",\"uuid\":\"5e30be34-c1af-4919-9af8-d4df8145ecd1\"}],\"packageUris\":[\"http://schema.mathworks.com/mf0/Connector/R2020b\"],\"version\":\"1.0\"}"
  Bus Element Out1 : Outport  PortName=envStatus
  Bus Element Out4 : Outport  Port=2  PortName=bayStatus
  wires:
  GravityCompensatorArray/1(envStatus) -> Bus Element Out1/1
  Bus Element In3/1 -> GravityCompensatorArray/1(ambientGravity)
  FusionPowerPlant/1(statusPower) -> ServicesController/3(statusPower)
  ConveyorNetwork/1(statusTransport) -> ServicesController/2(statusTransport)
  ServicesController/1(bayDirective) -> FusionPowerPlant/1(directive)
  Bus Element In2/1 -> ServicesController/1(directive)
  ServicesController/2(bayStatus) -> Bus Element Out4/1
  Bus Element In4/1 -> ConveyorNetwork/1(transportDirective)

== system PhysicalHyperCook/PrepBay ==
  Bus Element In1 : Inport  PortName=directive
  Bus Element In2 : Inport  Port=2  PortName=stagedCold
  Bus Element In3 : Inport  Port=3  PortName=stagedAmbient
  PrepController : Subsystem
      settings: PortSchema="{\"entries\":[{\"content\":{\"headerSize\":26,\"margin\":15,\"minimumSpacing\":25,\"sides\":[{\"content\":{\"connectorIds\":[\"In1\",\"In2\",\"In3\"]},\"type\":\"ConnectorPlacement.EquallySpacedRectSide\",\"uuid\":\"0731d988-4a26-4db6-8347-b78d2aa6954f\"},{\"content\":{\"connectorIds\":[\"Out1\",\"Out2\"],\"side\":\"RIGHT\"},\"type\":\"ConnectorPlacement.EquallySpacedRectSide\",\"uuid\":\"6e8ac7ed-a816-4c7e-8f31-c61224c9ac03\"},{\"content\":{\"side\":\"TOP\"},\"type\":\"ConnectorPlacement.EquallySpacedRectSide\",\"uuid\":\"7c48a918-2743-4697-bc21-ce4fb8bbcea2\"}]},\"type\":\"ConnectorPlacement.EquallySpacedConnector\",\"uuid\":\"5e30be34-c1af-4919-9af8-d4df8145ecd1\"}],\"packageUris\":[\"http://schema.mathworks.com/mf0/Connector/R2020b\"],\"version\":\"1.0\"}"
  RoboticPrepLine1 : Subsystem
      settings: PortSchema="{\"entries\":[{\"content\":{\"headerSize\":26,\"margin\":15,\"minimumSpacing\":25,\"sides\":[{\"content\":{\"connectorIds\":[\"In1\",\"In2\"]},\"type\":\"ConnectorPlacement.EquallySpacedRectSide\",\"uuid\":\"f830f98a-8e8b-4468-adf4-d6eab644987f\"},{\"content\":{\"connectorIds\":[\"Out1\",\"Out2\"],\"side\":\"RIGHT\"},\"type\":\"ConnectorPlacement.EquallySpacedRectSide\",\"uuid\":\"7e0d0116-b3ba-4668-b638-30d0f54ba087\"},{\"content\":{\"side\":\"TOP\"},\"type\":\"ConnectorPlacement.EquallySpacedRectSide\",\"uuid\":\"7b4146d3-46d2-45ca-8c34-b106f0d8cedd\"}]},\"type\":\"ConnectorPlacement.EquallySpacedConnector\",\"uuid\":\"3d911b2d-a78f-42ea-b869-5e09982d9f54\"}],\"packageUris\":[\"http://schema.mathworks.com/mf0/Connector/R2020b\"],\"version\":\"1.0\"}"
  RoboticPrepLine2 : Subsystem
      settings: PortSchema="{\"entries\":[{\"content\":{\"headerSize\":26,\"margin\":15,\"minimumSpacing\":25,\"sides\":[{\"content\":{\"connectorIds\":[\"In1\",\"In2\"]},\"type\":\"ConnectorPlacement.EquallySpacedRectSide\",\"uuid\":\"f830f98a-8e8b-4468-adf4-d6eab644987f\"},{\"content\":{\"connectorIds\":[\"Out1\",\"Out2\"],\"side\":\"RIGHT\"},\"type\":\"ConnectorPlacement.EquallySpacedRectSide\",\"uuid\":\"7e0d0116-b3ba-4668-b638-30d0f54ba087\"},{\"content\":{\"side\":\"TOP\"},\"type\":\"ConnectorPlacement.EquallySpacedRectSide\",\"uuid\":\"7b4146d3-46d2-45ca-8c34-b106f0d8cedd\"}]},\"type\":\"ConnectorPlacement.EquallySpacedConnector\",\"uuid\":\"3d911b2d-a78f-42ea-b869-5e09982d9f54\"}],\"packageUris\":[\"http://schema.mathworks.com/mf0/Connector/R2020b\"],\"version\":\"1.0\"}"
  Bus Element Out1 : Outport  PortName=preppedBatch1
  Bus Element Out4 : Outport  Port=2  PortName=preppedBatch2
  Bus Element Out5 : Outport  Port=3  PortName=bayStatus
  wires:
  RoboticPrepLine1/2(statusPrep1) -> PrepController/2(statusPrep1)
  RoboticPrepLine2/2(statusPrep2) -> PrepController/3(statusPrep2)
  Bus Element In2/1 -> RoboticPrepLine1/1(stagedCold)
  RoboticPrepLine2/1(preppedBatch2) -> Bus Element Out4/1
  Bus Element In3/1 -> RoboticPrepLine2/1(stagedAmbient)
  RoboticPrepLine1/1(preppedBatch1) -> Bus Element Out1/1
  Bus Element In1/1 -> PrepController/1(directive)
  PrepController/1(bayDirective) -> RoboticPrepLine2/2(directive), RoboticPrepLine1/2(directive)
  PrepController/2(bayStatus) -> Bus Element Out5/1

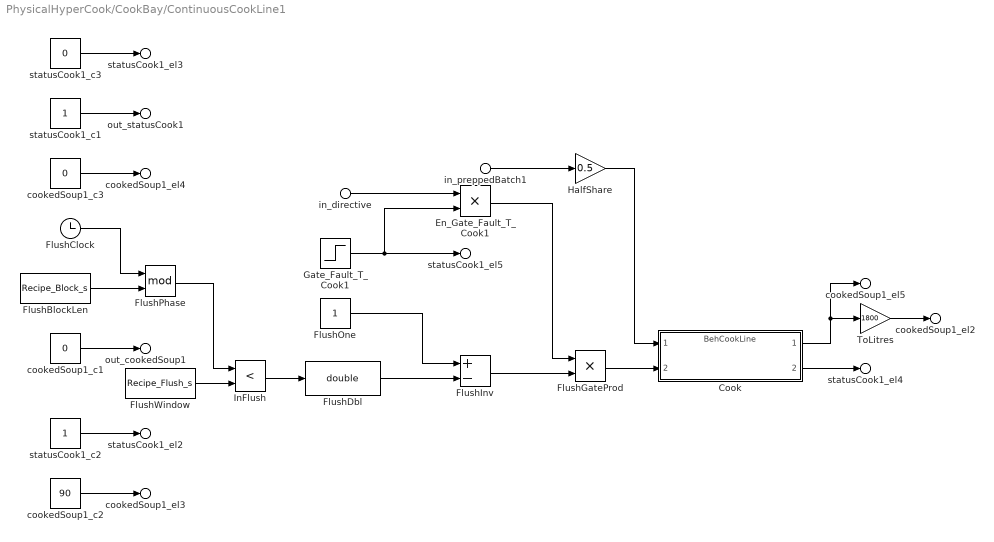
== system PhysicalHyperCook/CookBay/ContinuousCookLine1 ==
  in_preppedBatch1 : Inport  PortName=preppedBatch1  Element=flow_bps
  in_directive : Inport  Port=2  PortName=directive  Element=setpoint
  Cook : ModelReference  ModelNameDialog=BehCookLine  UsingDefaultArgumentValue=0,0,0,0  SimulationMode=Normal  ModelReferenceVersion=1.5
  En_Gate_Fault_T_Cook1 : Product
  FlushBlockLen : Constant  Value=Recipe_Block_s
  FlushClock : Clock
  FlushDbl : DataTypeConversion  OutDataTypeStr=double  SaturateOnIntegerOverflow=off  RndMeth=Floor
  FlushGateProd : Product
  FlushInv : Sum  Inputs=+-
  FlushOne : Constant
  FlushPhase : Math  Operator=mod
  FlushWindow : Constant  Value=Recipe_Flush_s
  Gate_Fault_T_Cook1 : Step  Time=Fault_T_Cook1  InitialValue=1  FinalValue=0  SampleTime=0
  HalfShare : Gain  Gain=0.5
  InFlush : RelationalOperator  Operator=<  OutDataTypeStr=boolean  RndMeth=Simplest  InputSameDT=off
  ToLitres : Gain  Gain=1800
  cookedSoup1_c1 : Constant  Value=0
  cookedSoup1_c2 : Constant  Value=90
  cookedSoup1_c3 : Constant  Value=0
  statusCook1_c1 : Constant
  statusCook1_c2 : Constant
  statusCook1_c3 : Constant  Value=0
  out_cookedSoup1 : Outport  PortName=cookedSoup1  Element=batchId
  cookedSoup1_el2 : Outport  PortName=cookedSoup1  Element=volume_L
  cookedSoup1_el3 : Outport  PortName=cookedSoup1  Element=temp_C
  cookedSoup1_el4 : Outport  PortName=cookedSoup1  Element=contamination_ppm
  cookedSoup1_el5 : Outport  PortName=cookedSoup1  Element=flow_bps
  out_statusCook1 : Outport  Port=2  PortName=statusCook1  Element=unitId
  statusCook1_el2 : Outport  Port=2  PortName=statusCook1  Element=opState
  statusCook1_el3 : Outport  Port=2  PortName=statusCook1  Element=faultCode
  statusCook1_el4 : Outport  Port=2  PortName=statusCook1  Element=power_kW
  statusCook1_el5 : Outport  Port=2  PortName=statusCook1  Element=health
  wires:
  statusCook1_c1/1 -> out_statusCook1/1
  statusCook1_c3/1 -> statusCook1_el3/1
  cookedSoup1_c1/1 -> out_cookedSoup1/1
  cookedSoup1_c3/1 -> cookedSoup1_el4/1
  FlushBlockLen/1 -> FlushPhase/2
  FlushClock/1 -> FlushPhase/1
  statusCook1_c2/1 -> statusCook1_el2/1
  ToLitres/1 -> cookedSoup1_el2/1
  cookedSoup1_c2/1 -> cookedSoup1_el3/1
  HalfShare/1 -> Cook/1
  FlushPhase/1 -> InFlush/1
  Cook/2 -> statusCook1_el4/1
  FlushWindow/1 -> InFlush/2
  InFlush/1 -> FlushDbl/1
  in_directive/1 -> En_Gate_Fault_T_Cook1/1
  Gate_Fault_T_Cook1/1 -> En_Gate_Fault_T_Cook1/2, statusCook1_el5/1
  FlushGateProd/1 -> Cook/2
  FlushOne/1 -> FlushInv/1
  FlushDbl/1 -> FlushInv/2
  in_preppedBatch1/1 -> HalfShare/1
  En_Gate_Fault_T_Cook1/1 -> FlushGateProd/1
  FlushInv/1 -> FlushGateProd/2
  Cook/1 -> cookedSoup1_el5/1, ToLitres/1

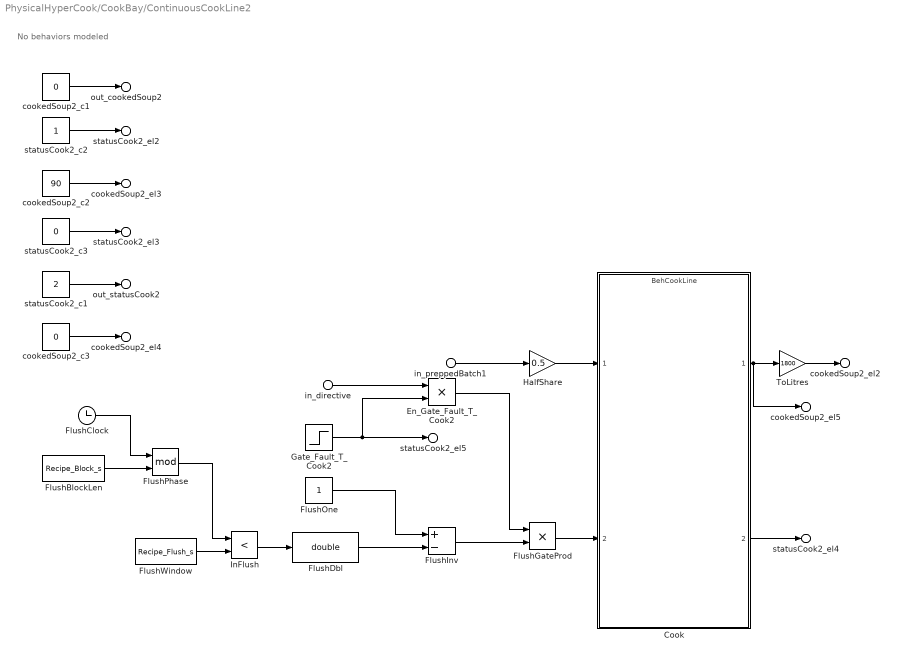
== system PhysicalHyperCook/CookBay/ContinuousCookLine2 ==
  note: No behaviors modeled
  in_preppedBatch1 : Inport  PortName=preppedBatch1  Element=flow_bps
  in_directive : Inport  Port=2  PortName=directive  Element=setpoint
  Cook : ModelReference  ModelNameDialog=BehCookLine  UsingDefaultArgumentValue=0,0,0,0  SimulationMode=Normal  ModelReferenceVersion=1.5
  En_Gate_Fault_T_Cook2 : Product
  FlushBlockLen : Constant  Value=Recipe_Block_s
  FlushClock : Clock
  FlushDbl : DataTypeConversion  OutDataTypeStr=double  SaturateOnIntegerOverflow=off  RndMeth=Floor
  FlushGateProd : Product
  FlushInv : Sum  Inputs=+-
  FlushOne : Constant
  FlushPhase : Math  Operator=mod
  FlushWindow : Constant  Value=Recipe_Flush_s
  Gate_Fault_T_Cook2 : Step  Time=Fault_T_Cook2  InitialValue=1  FinalValue=0  SampleTime=0
  HalfShare : Gain  Gain=0.5
  InFlush : RelationalOperator  Operator=<  OutDataTypeStr=boolean  RndMeth=Simplest  InputSameDT=off
  ToLitres : Gain  Gain=1800
  cookedSoup2_c1 : Constant  Value=0
  cookedSoup2_c2 : Constant  Value=90
  cookedSoup2_c3 : Constant  Value=0
  statusCook2_c1 : Constant  Value=2
  statusCook2_c2 : Constant
  statusCook2_c3 : Constant  Value=0
  out_cookedSoup2 : Outport  PortName=cookedSoup2  Element=batchId
  cookedSoup2_el2 : Outport  PortName=cookedSoup2  Element=volume_L
  cookedSoup2_el3 : Outport  PortName=cookedSoup2  Element=temp_C
  cookedSoup2_el4 : Outport  PortName=cookedSoup2  Element=contamination_ppm
  cookedSoup2_el5 : Outport  PortName=cookedSoup2  Element=flow_bps
  out_statusCook2 : Outport  Port=2  PortName=statusCook2  Element=unitId
  statusCook2_el2 : Outport  Port=2  PortName=statusCook2  Element=opState
  statusCook2_el3 : Outport  Port=2  PortName=statusCook2  Element=faultCode
  statusCook2_el4 : Outport  Port=2  PortName=statusCook2  Element=power_kW
  statusCook2_el5 : Outport  Port=2  PortName=statusCook2  Element=health
  wires:
  cookedSoup2_c1/1 -> out_cookedSoup2/1
  cookedSoup2_c3/1 -> cookedSoup2_el4/1
  statusCook2_c1/1 -> out_statusCook2/1
  statusCook2_c3/1 -> statusCook2_el3/1
  FlushBlockLen/1 -> FlushPhase/2
  HalfShare/1 -> Cook/1
  FlushClock/1 -> FlushPhase/1
  ToLitres/1 -> cookedSoup2_el2/1
  cookedSoup2_c2/1 -> cookedSoup2_el3/1
  statusCook2_c2/1 -> statusCook2_el2/1
  FlushInv/1 -> FlushGateProd/2
  FlushPhase/1 -> InFlush/1
  FlushWindow/1 -> InFlush/2
  InFlush/1 -> FlushDbl/1
  in_directive/1 -> En_Gate_Fault_T_Cook2/1
  Gate_Fault_T_Cook2/1 -> En_Gate_Fault_T_Cook2/2, statusCook2_el5/1
  FlushOne/1 -> FlushInv/1
  FlushDbl/1 -> FlushInv/2
  in_preppedBatch1/1 -> HalfShare/1
  En_Gate_Fault_T_Cook2/1 -> FlushGateProd/1
  FlushGateProd/1 -> Cook/2
  Cook/1 -> cookedSoup2_el5/1, ToLitres/1
  Cook/2 -> statusCook2_el4/1

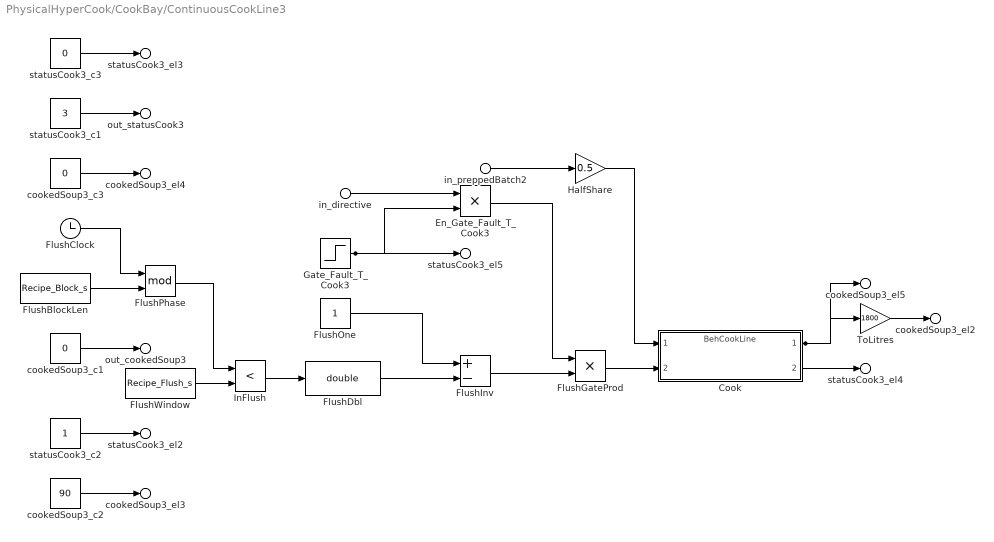
== system PhysicalHyperCook/CookBay/ContinuousCookLine3 ==
  in_preppedBatch2 : Inport  PortName=preppedBatch2  Element=flow_bps
  in_directive : Inport  Port=2  PortName=directive  Element=setpoint
  Cook : ModelReference  ModelNameDialog=BehCookLine  UsingDefaultArgumentValue=0,0,0,0  SimulationMode=Normal  ModelReferenceVersion=1.5
  En_Gate_Fault_T_Cook3 : Product
  FlushBlockLen : Constant  Value=Recipe_Block_s
  FlushClock : Clock
  FlushDbl : DataTypeConversion  OutDataTypeStr=double  SaturateOnIntegerOverflow=off  RndMeth=Floor
  FlushGateProd : Product
  FlushInv : Sum  Inputs=+-
  FlushOne : Constant
  FlushPhase : Math  Operator=mod
  FlushWindow : Constant  Value=Recipe_Flush_s
  Gate_Fault_T_Cook3 : Step  Time=Fault_T_Cook3  InitialValue=1  FinalValue=0  SampleTime=0
  HalfShare : Gain  Gain=0.5
  InFlush : RelationalOperator  Operator=<  OutDataTypeStr=boolean  RndMeth=Simplest  InputSameDT=off
  ToLitres : Gain  Gain=1800
  cookedSoup3_c1 : Constant  Value=0
  cookedSoup3_c2 : Constant  Value=90
  cookedSoup3_c3 : Constant  Value=0
  statusCook3_c1 : Constant  Value=3
  statusCook3_c2 : Constant
  statusCook3_c3 : Constant  Value=0
  out_cookedSoup3 : Outport  PortName=cookedSoup3  Element=batchId
  cookedSoup3_el2 : Outport  PortName=cookedSoup3  Element=volume_L
  cookedSoup3_el3 : Outport  PortName=cookedSoup3  Element=temp_C
  cookedSoup3_el4 : Outport  PortName=cookedSoup3  Element=contamination_ppm
  cookedSoup3_el5 : Outport  PortName=cookedSoup3  Element=flow_bps
  out_statusCook3 : Outport  Port=2  PortName=statusCook3  Element=unitId
  statusCook3_el2 : Outport  Port=2  PortName=statusCook3  Element=opState
  statusCook3_el3 : Outport  Port=2  PortName=statusCook3  Element=faultCode
  statusCook3_el4 : Outport  Port=2  PortName=statusCook3  Element=power_kW
  statusCook3_el5 : Outport  Port=2  PortName=statusCook3  Element=health
  wires:
  Gate_Fault_T_Cook3/1 -> En_Gate_Fault_T_Cook3/2, statusCook3_el5/1
  statusCook3_c3/1 -> statusCook3_el3/1
  statusCook3_c1/1 -> out_statusCook3/1
  FlushBlockLen/1 -> FlushPhase/2
  cookedSoup3_c1/1 -> out_cookedSoup3/1
  FlushClock/1 -> FlushPhase/1
  cookedSoup3_c3/1 -> cookedSoup3_el4/1
  statusCook3_c2/1 -> statusCook3_el2/1
  ToLitres/1 -> cookedSoup3_el2/1
  cookedSoup3_c2/1 -> cookedSoup3_el3/1
  FlushInv/1 -> FlushGateProd/2
  FlushPhase/1 -> InFlush/1
  FlushWindow/1 -> InFlush/2
  InFlush/1 -> FlushDbl/1
  in_directive/1 -> En_Gate_Fault_T_Cook3/1
  FlushOne/1 -> FlushInv/1
  in_preppedBatch2/1 -> HalfShare/1
  FlushDbl/1 -> FlushInv/2
  En_Gate_Fault_T_Cook3/1 -> FlushGateProd/1
  HalfShare/1 -> Cook/1
  FlushGateProd/1 -> Cook/2
  Cook/1 -> cookedSoup3_el5/1, ToLitres/1
  Cook/2 -> statusCook3_el4/1

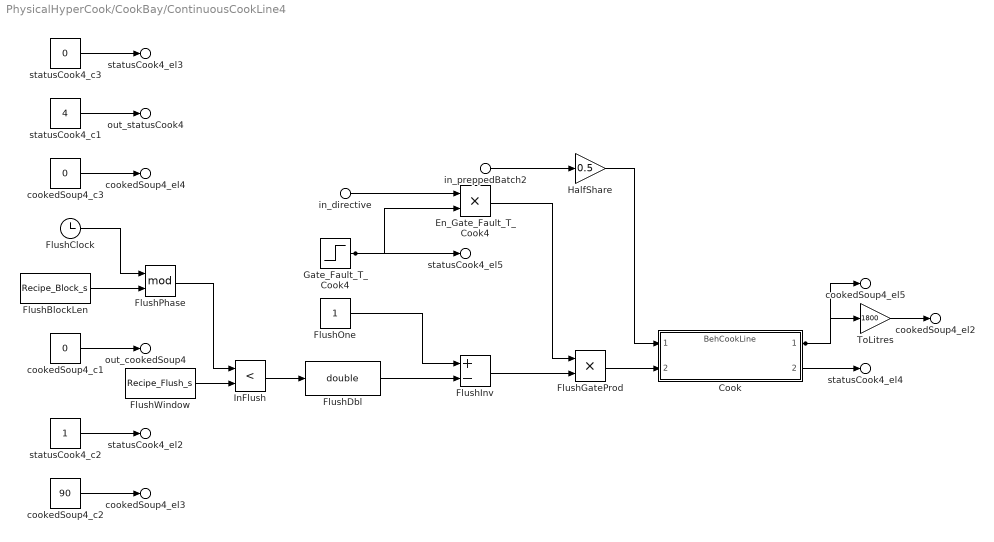
== system PhysicalHyperCook/CookBay/ContinuousCookLine4 ==
  in_preppedBatch2 : Inport  PortName=preppedBatch2  Element=flow_bps
  in_directive : Inport  Port=2  PortName=directive  Element=setpoint
  Cook : ModelReference  ModelNameDialog=BehCookLine  UsingDefaultArgumentValue=0,0,0,0  SimulationMode=Normal  ModelReferenceVersion=1.5
  En_Gate_Fault_T_Cook4 : Product
  FlushBlockLen : Constant  Value=Recipe_Block_s
  FlushClock : Clock
  FlushDbl : DataTypeConversion  OutDataTypeStr=double  SaturateOnIntegerOverflow=off  RndMeth=Floor
  FlushGateProd : Product
  FlushInv : Sum  Inputs=+-
  FlushOne : Constant
  FlushPhase : Math  Operator=mod
  FlushWindow : Constant  Value=Recipe_Flush_s
  Gate_Fault_T_Cook4 : Step  Time=Fault_T_Cook4  InitialValue=1  FinalValue=0  SampleTime=0
  HalfShare : Gain  Gain=0.5
  InFlush : RelationalOperator  Operator=<  OutDataTypeStr=boolean  RndMeth=Simplest  InputSameDT=off
  ToLitres : Gain  Gain=1800
  cookedSoup4_c1 : Constant  Value=0
  cookedSoup4_c2 : Constant  Value=90
  cookedSoup4_c3 : Constant  Value=0
  statusCook4_c1 : Constant  Value=4
  statusCook4_c2 : Constant
  statusCook4_c3 : Constant  Value=0
  out_cookedSoup4 : Outport  PortName=cookedSoup4  Element=batchId
  cookedSoup4_el2 : Outport  PortName=cookedSoup4  Element=volume_L
  cookedSoup4_el3 : Outport  PortName=cookedSoup4  Element=temp_C
  cookedSoup4_el4 : Outport  PortName=cookedSoup4  Element=contamination_ppm
  cookedSoup4_el5 : Outport  PortName=cookedSoup4  Element=flow_bps
  out_statusCook4 : Outport  Port=2  PortName=statusCook4  Element=unitId
  statusCook4_el2 : Outport  Port=2  PortName=statusCook4  Element=opState
  statusCook4_el3 : Outport  Port=2  PortName=statusCook4  Element=faultCode
  statusCook4_el4 : Outport  Port=2  PortName=statusCook4  Element=power_kW
  statusCook4_el5 : Outport  Port=2  PortName=statusCook4  Element=health
  wires:
  FlushClock/1 -> FlushPhase/1
  cookedSoup4_c3/1 -> cookedSoup4_el4/1
  statusCook4_c3/1 -> statusCook4_el3/1
  Gate_Fault_T_Cook4/1 -> statusCook4_el5/1, En_Gate_Fault_T_Cook4/2
  statusCook4_c1/1 -> out_statusCook4/1
  FlushBlockLen/1 -> FlushPhase/2
  En_Gate_Fault_T_Cook4/1 -> FlushGateProd/1
  cookedSoup4_c1/1 -> out_cookedSoup4/1
  statusCook4_c2/1 -> statusCook4_el2/1
  cookedSoup4_c2/1 -> cookedSoup4_el3/1
  FlushPhase/1 -> InFlush/1
  FlushWindow/1 -> InFlush/2
  InFlush/1 -> FlushDbl/1
  HalfShare/1 -> Cook/1
  FlushInv/1 -> FlushGateProd/2
  in_directive/1 -> En_Gate_Fault_T_Cook4/1
  FlushOne/1 -> FlushInv/1
  FlushDbl/1 -> FlushInv/2
  in_preppedBatch2/1 -> HalfShare/1
  FlushGateProd/1 -> Cook/2
  Cook/1 -> ToLitres/1, cookedSoup4_el5/1
  Cook/2 -> statusCook4_el4/1
  ToLitres/1 -> cookedSoup4_el2/1
